simulink model "JointSpaceInverseDynamics"  (R2023a)
settings: Solver=VariableStepAuto  StartTime=0.0  StopTime=3  RelTol=1e-3
values from neighbouring files (symbols this model uses):
  Kd = [[70,0,0] ... (first row only)    [parameters.m]
  Kp = [[200,0,0] ... (first row only)    [parameters.m]
libraries: robotcorelib x1
settings Model: Creator=uzair  LastModifiedBy=syedj
settings OptimizationCC: ReuseModelBlockBuffer=off

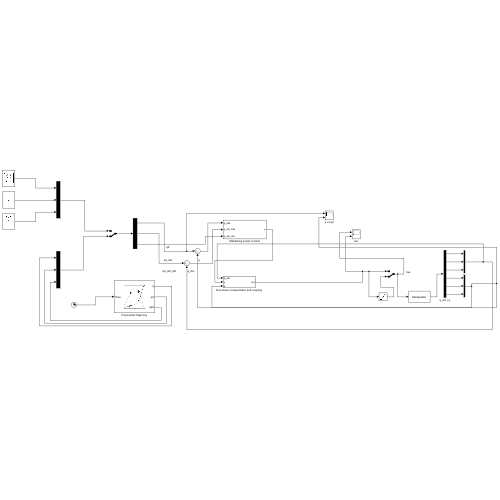
[thumbnail: Simulink's stored preview of the top-level diagram]
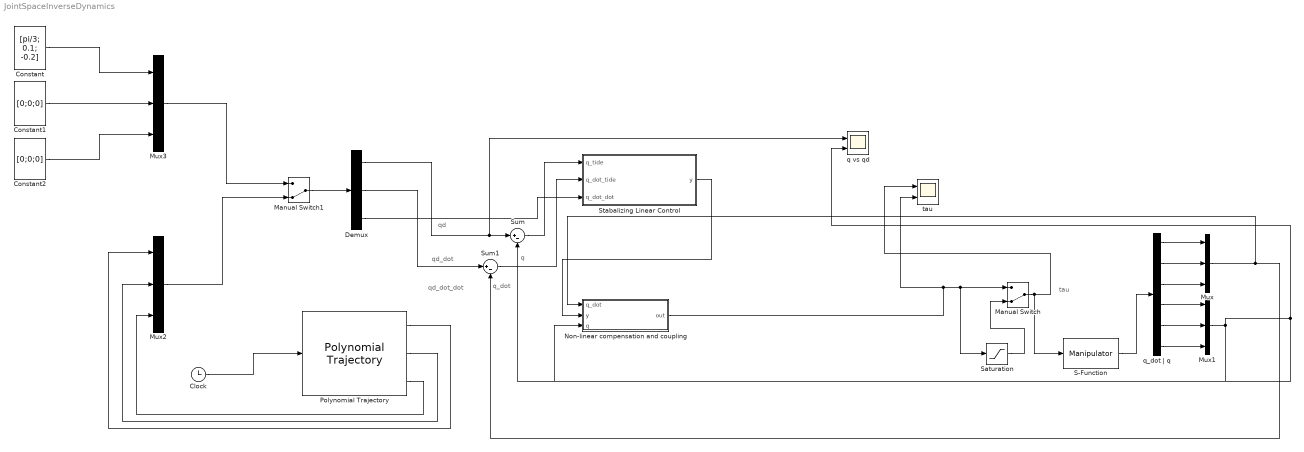
== system JointSpaceInverseDynamics ==
  note: qd_dot_dot
  note: qd_dot
  note: qd
  note: q
  note: tau
  note: q_dot
  Clock : Clock
  Constant : Constant  Value=[pi/3; 0.1; -0.2]  VectorParams1D=off
  Constant1 : Constant  Value=[0;0;0]  VectorParams1D=off
  Constant2 : Constant  Value=[0;0;0]  VectorParams1D=off
  Demux : Demux  Outputs=3
  Manual Switch : ManualSwitch  CurrentSetting=0
  Manual Switch1 : ManualSwitch  CurrentSetting=0
  Mux{,1..3} (4 alike) : Mux  Inputs=3
  Non-linear compensation and coupling : Subsystem
  Polynomial Trajectory : robotcorelib/Polynomial Trajectory  WaypointSource=Internal  Waypoints=[pi,-pi,pi,-pi; -2,2,-2,2; -pi,pi,-pi,pi]  TimePoints=[0,1, 2, 3 ]  TimeInterval=[ 1, 4 ]  Method=Cubic Polynomial  ParameterSource=Internal  VelocityBoundaryCondition=zeros( 3,4 )  AccelerationBoundaryCondition=zeros( 3,3 )  SimulateUsing=Interpreted execution
  S-Function : S-Function  FunctionName=Manipulator  Parameters=params  SFunctionDeploymentMode=off  EnableBusSupport=off
  Saturation : Saturate  UpperLimit=100  LowerLimit=-100
  Stabalizing Linear Control : Subsystem
  Sum : Sum  Inputs=|+-
  Sum1 : Sum  Inputs=|+-
  q vs qd : Scope  NumInputPorts=2
  q_dot | q : Demux  Outputs=6
  tau : Scope  NumInputPorts=2
  wires:
  Stabalizing Linear Control/1(y) -> Non-linear compensation and coupling/2(y)
  S-Function/1 -> q_dot | q/1
  q_dot | q/1 -> Mux/1
  q_dot | q/2 -> Mux/2
  q_dot | q/3 -> Mux/3
  q_dot | q/6 -> Mux1/3
  q_dot | q/5 -> Mux1/2
  q_dot | q/4 -> Mux1/1
  Mux/1 -> Non-linear compensation and coupling/1(q_dot), Sum1/2
  Mux1/1 -> q vs qd/2, Non-linear compensation and coupling/3(q), Sum/2
  Sum/1 -> Stabalizing Linear Control/1(q_tide)
  Sum1/1 -> Stabalizing Linear Control/2(q_dot_tide)
  Clock/1 -> Polynomial Trajectory/1
  Manual Switch/1 -> S-Function/1, tau/1
  Non-linear compensation and coupling/1(out) -> tau/2, Saturation/1, Manual Switch/1
  Polynomial Trajectory/1 -> Mux2/1
  Polynomial Trajectory/2 -> Mux2/2
  Polynomial Trajectory/3 -> Mux2/3
  Constant/1 -> Mux3/1
  Constant1/1 -> Mux3/2
  Constant2/1 -> Mux3/3
  Mux3/1 -> Manual Switch1/1
  Mux2/1 -> Manual Switch1/2
  Manual Switch1/1 -> Demux/1
  Demux/1 -> q vs qd/1, Sum/1
  Demux/2 -> Sum1/1
  Demux/3 -> Stabalizing Linear Control/3(q_dot_dot)
  Saturation/1 -> Manual Switch/2

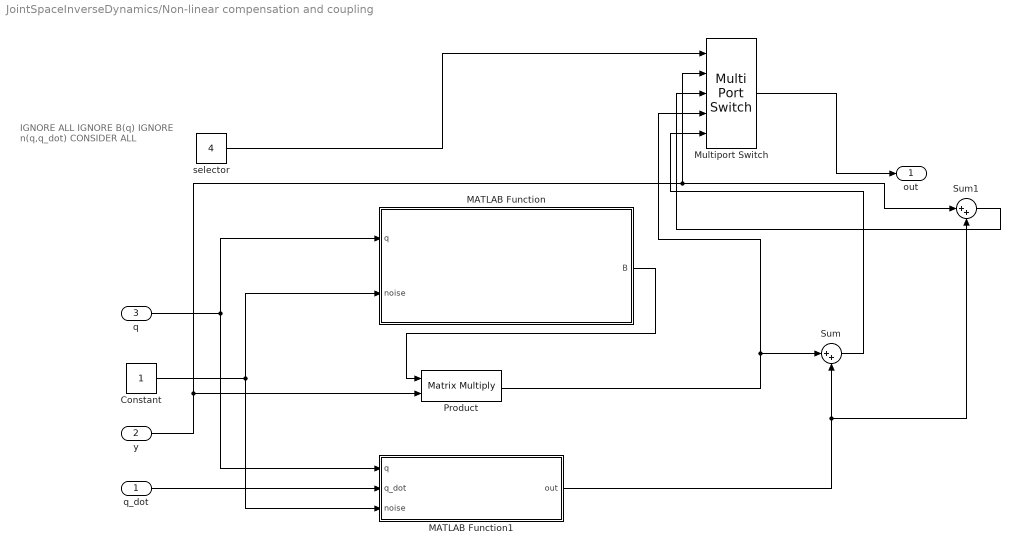
== system JointSpaceInverseDynamics/Non-linear compensation and coupling ==
  note: IGNORE ALL
      | IGNORE B(q)
      | IGNORE n(q,q_dot)
      | CONSIDER ALL
  q_dot : Inport
  y : Inport  Port=2
  q : Inport  Port=3
  Constant : Constant
  MATLAB Function : MATLAB Function  TreatAsAtomicUnit=on
  MATLAB Function1 : MATLAB Function  TreatAsAtomicUnit=on
  Multiport Switch : MultiPortSwitch  Inputs=4  SaturateOnIntegerOverflow=off  InputSameDT=off
  Product : Product  Multiplication=Matrix(*)
  Sum : Sum  Inputs=|++
  Sum1 : Sum  Inputs=|++
  selector : Constant  Value=4
  out : Outport
  wires:
  q/1 -> MATLAB Function1/1(q), MATLAB Function/1(q)
  MATLAB Function/1(B) -> Product/1
  y/1 -> Sum1/1, Multiport Switch/2, Product/2
  Product/1 -> Multiport Switch/4, Sum/1
  q_dot/1 -> MATLAB Function1/2(q_dot)
  MATLAB Function1/1(out) -> Sum1/2, Sum/2
  Constant/1 -> MATLAB Function1/3(noise), MATLAB Function/2(noise)
  selector/1 -> Multiport Switch/1
  Multiport Switch/1 -> out/1
  Sum1/1 -> Multiport Switch/3
  Sum/1 -> Multiport Switch/5

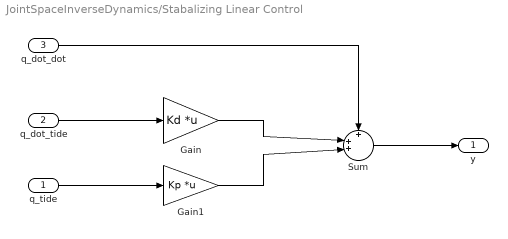
== system JointSpaceInverseDynamics/Stabalizing Linear Control ==
  q_tide : Inport
  q_dot_tide : Inport  Port=2
  q_dot_dot : Inport  Port=3
  Gain : Gain  Gain=Kd  Multiplication=Matrix(K*u)
  Gain1 : Gain  Gain=Kp  Multiplication=Matrix(K*u)
  Sum : Sum  Inputs=+|++||
  y : Outport
  wires:
  q_tide/1 -> Gain1/1
  q_dot_dot/1 -> Sum/1
  Gain1/1 -> Sum/3
  Sum/1 -> y/1
  q_dot_tide/1 -> Gain/1
  Gain/1 -> Sum/2

== matlab function JointSpaceInverseDynamics/Non-linear compensation and coupling/MATLAB Function1 ==
  data: q input; out output; q_dot input; params parameter; noise input
function out = n(q, q_dot, params, noise)
    
    m1 = params.m(1) * noise;
    m2 = params.m(2) * noise;
    m3 = params.m(3) * noise;

    q1 = q(1);
    q2 = q(2);
    q3 = q(3);

    q1_dot = q_dot(1);
    q2_dot = q_dot(2);
    q3_dot = q_dot(3);

    g = params.g;

    Fv = params.Fv;

    a1 = 0.02;
    a2 = 0.03;
    a3 = 0.01;
    b1 = 0.1256;
    b2 = 0.03;
    b3 = 0.01;
    c1 = 0.4;
    c2 = 0.46;
    c3 = 0.15;
 
    B = [[(a2^2*m2)/12 + (3*a1^4*m1)/2 + (a3^2*m3)/12 + (3*b1^4*m1)/2 + (b3^2*m3)/12 + c1^2*m1 + c1^2*m2 + c1^2*m3 + (7*c2^2*m2)/12 + (c3^2*m3)/2 + m3*q3^2 + 3*a1^2*b1^2*m1 - c1*c2*m2 + c1*c3*m3 + 2*c1*m3*q3 + c3*m3*q3,       0,  0]
[                                                                                                                                                                                                               0, m2 + m3,  0]
[                                                                                                                                                                                                               0,       0, m3]];

    C = [[ (m3*q3_dot*(2*c1 + c3 + 2*q3))/2, 0, (m3*q1_dot*(2*c1 + c3 + 2*q3))/2]
[                                0, 0,                                0]
[-(m3*q1_dot*(2*c1 + c3 + 2*q3))/2, 0,                                0]];


G = [(c1*g*m1*cos(q1))/2 + g*m2*cos(q1)*(c1 - c2/2) + g*m3*cos(q1)*(c1 + c3/2 + q3)
        0;
        g*m3*sin(q1)];



    out = C*q_dot + diag(Fv)*q_dot + G;
end

== matlab function JointSpaceInverseDynamics/Non-linear compensation and coupling/MATLAB Function ==
  data: q input; B output; params parameter; noise input
function B = inertiaMatrix(q, params, noise)
    q1 = q(1);
    q2 = q(2);
    q3 = q(3);

    m1 = params.m(1) * noise;
    m2 = params.m(2) * noise;
    m3 = params.m(3) * noise;

    a1 = 0.02;
    a2 = 0.03;
    a3 = 0.01;
    b1 = 0.1256;
    b2 = 0.03;
    b3 = 0.01;
    c1 = 0.4;
    c2 = 0.46;
    c3 = 0.15;

    B = [[(a2^2*m2)/12 + (3*a1^4*m1)/2 + (a3^2*m3)/12 + (3*b1^4*m1)/2 + (b3^2*m3)/12 + c1^2*m1 + c1^2*m2 + c1^2*m3 + (7*c2^2*m2)/12 + (c3^2*m3)/2 + m3*q3^2 + 3*a1^2*b1^2*m1 - c1*c2*m2 + c1*c3*m3 + 2*c1*m3*q3 + c3*m3*q3,       0,  0]
[                                                                                                                                                                                                               0, m2 + m3,  0]
[                                                                                                                                                                                                               0,       0, m3]];


end
